simulink model "Simscape_Benchmark_Model"  (R2020b)
settings: Solver=ode45  StartTime=0.0  StopTime=10.0  RelTol=1e-8  AbsTol=1e-9
undefined symbols (not defined in the file): Bus, FSM, ISOL, Model, PMA, RWIsol, RWS, SA, SADM, slosh, X, Y, Z
libraries: sm_lib x159, nesl_utility x85, simulink x4
(part 5 of 6)

== system Simscape_Benchmark_Model/WEMS + Reaction wheels/RW saturation and friction model ==
  note: 1) Add Subsystem or Model blocks as valid variant choices.
      | 2) You cannot connect blocks at this level. At simulation, connectivity is automatically
      | determined, based on the active variant and port name matching.
  In1 : Inport
  No saturations - No friction model : Subsystem  VariantControl=Benchmark.config.status.RWS_Sat==0 && Benchmark.config.status.RWS_Fric==0 && Benchmark.config.status.RWS_Frict_spikes==0
  Saturations +  friction model : Subsystem  VariantControl=Benchmark.config.status.RWS_Sat==1 && Benchmark.config.status.RWS_Fric==1 && Benchmark.config.status.RWS_Frict_spikes==0
  Saturations + friction model + friction spikes : Subsystem  VariantControl=Benchmark.config.status.RWS_Sat==1 && Benchmark.config.status.RWS_Fric==1 && Benchmark.config.status.RWS_Frict_spikes==1
  Saturations - No friction model : Subsystem  VariantControl=Benchmark.config.status.RWS_Sat==1 && Benchmark.config.status.RWS_Fric==0 && Benchmark.config.status.RWS_Frict_spikes==0
  Out1 : Outport

== system Simscape_Benchmark_Model/WEMS + Reaction wheels/RWS ==
  note: 1) Add Subsystem or Model blocks as valid variant choices.
      | 2) You cannot connect blocks at this level. At simulation, connectivity is automatically
      | determined, based on the active variant and port name matching.
  Balanced RWS : Subsystem  VariantControl="Benchmark.config.status.RWS_Harmdist==   0"
  RWS with disturbance harmonics : Subsystem  VariantControl="Benchmark.config.status.RWS_Harmdist==   1"
  Connection Port : PMIOPort  Tag=PMCPort  Side=Left
  Connection Port1 : PMIOPort  Tag=PMCPort  Port=2  Side=Left
  Connection Port2 : PMIOPort  Tag=PMCPort  Port=3  Side=Left
  Connection Port3 : PMIOPort  Tag=PMCPort  Port=4  Side=Left

== system Simscape_Benchmark_Model/WEMS + Reaction wheels/RW saturation and friction model/No saturations - No friction model ==
  In1 : Inport
  Out1 : Outport
  wires:
  In1/1 -> Out1/1

== system Simscape_Benchmark_Model/WEMS + Reaction wheels/RW saturation and friction model/Saturations +  friction model ==
  In1 : Inport
  RW friction model : Subsystem
  Terminator2 : Terminator
  sat_max_torque : Saturate  UpperLimit=RWS.max_torque  LowerLimit=-RWS.max_torque
  Out1 : Outport
  wires:
  In1/1 -> sat_max_torque/1
  sat_max_torque/1 -> RW friction model/1(Trq_cmd_rw)
  RW friction model/1(Torque_RW) -> Out1/1
  RW friction model/2(RW_TRQfriction) -> Terminator2/1

== system Simscape_Benchmark_Model/WEMS + Reaction wheels/RW saturation and friction model/Saturations + friction model + friction spikes ==
  In1 : Inport
  Gain : Gain  Gain=-1
  Mux : Mux
  Product : Product
  RW friction model : Subsystem
  Rate Transition : RateTransition  OutPortSampleTime=Model.ACS_sampling.Ts
  Spike generation RW1 : Subsystem
  Spike generation RW2 : Subsystem
  Spike generation RW3 : Subsystem
  Spike generation RW4 : Subsystem
  Sum : Sum
  Terminator2 : Terminator
  sat_max_torque : Saturate  UpperLimit=RWS.max_torque  LowerLimit=-RWS.max_torque
  Out1 : Outport
  tag scope: RW_torque_spikes=global
  wires:
  In1/1 -> sat_max_torque/1
  Sum/1 -> Out1/1
  Mux/1 -> Rate Transition/1
  RW friction model/1(Torque_RW) -> Sum/1
  RW friction model/2(RW_TRQfriction) -> Terminator2/1
  sat_max_torque/1 -> RW friction model/1(Trq_cmd_rw)
  Spike generation RW1/1(Out1) -> Mux/1
  Spike generation RW3/1(Out1) -> Mux/3
  Spike generation RW2/1(Out1) -> Mux/2
  Spike generation RW4/1(Out1) -> Mux/4
  RW friction model/3(sign_omega) -> Product/1
  Rate Transition/1 -> Gain/1
  Product/1 -> [RW_torque_spikes], Sum/2
  Gain/1 -> Product/2

== system Simscape_Benchmark_Model/WEMS + Reaction wheels/RW saturation and friction model/Saturations - No friction model ==
  In1 : Inport
  sat_max_torque : Saturate  UpperLimit=RWS.max_torque  LowerLimit=-RWS.max_torque
  Out1 : Outport
  wires:
  In1/1 -> sat_max_torque/1
  sat_max_torque/1 -> Out1/1

== system Simscape_Benchmark_Model/WEMS + Reaction wheels/RWS/Balanced RWS ==
  Cylindrical Solid{,1..3} (4 alike) : sm_lib/Body Elements/Cylindrical Solid  GraphicAmbientColor=[0.15 0.15 0.15 1.0]  BasedOnType=Density  CenterOfMass=[0 0 0]  CenterOfMassUnits=m  GraphicDiffuseColor=[0.8 0.0 0.0]  CylinderLength=0.1  CylinderLengthUnits=m  CylinderRadius=0.15  CylinderRadiusUnits=m  Density=1000  DensityUnits=kg/m^3  DoExposeReferenceFrame=on  GraphicEmissiveColor=[0.0 0.0 0.0 1.0]  ExportEntireGeometry=off  SerializedFrames=<Frames/>  MarkerShape=Sphere  MarkerSize=10  GraphicType=FromGeometry  InertiaType=Custom  Mass=RWS.m  MassUnits=kg  MomentsOfInertia=[RWS.Ir RWS.Ir RWS.Iw]  MomentsOfInertiaUnits=kg*m^2  GraphicOpacity=0.8  ProductsOfInertia=[0 0 0]  ProductsOfInertiaUnits=kg*m^2  GraphicShininess=75  GraphicSpecularColor=[0.5 0.5 0.5 1.0]  GraphicVisPropType=SimpleVisualProperties
  Frame R_RW{1..4} (4 alike) : sm_lib/Body Elements/Graphic  GraphicType=Marker  MarkerShape=Frame  MarkerSize=35  GraphicVisPropType=SimpleVisualProperties  GraphicDiffuseColor=[0.2 1.0 1.0]  GraphicSpecularColor=[0.5 0.5 0.5 1.0]  GraphicAmbientColor=[0.15 0.15 0.15 1.0]  GraphicEmissiveColor=[0.0 0.0 0.0 1.0]  GraphicShininess=75  GraphicOpacity=0.5
  Connection Port : PMIOPort  Tag=PMCPort  Side=Left
  Connection Port1 : PMIOPort  Tag=PMCPort  Port=2  Side=Left
  Connection Port2 : PMIOPort  Tag=PMCPort  Port=3  Side=Left
  Connection Port3 : PMIOPort  Tag=PMCPort  Port=4  Side=Left
  connections:
  Frame R_RW1/RConn1 -- Connection Port/RConn1 -- Cylindrical Solid/RConn1
  Cylindrical Solid1/RConn1 -- Connection Port1/RConn1 -- Frame R_RW2/RConn1
  Cylindrical Solid2/RConn1 -- Connection Port2/RConn1 -- Frame R_RW3/RConn1
  Cylindrical Solid3/RConn1 -- Connection Port3/RConn1 -- Frame R_RW4/RConn1

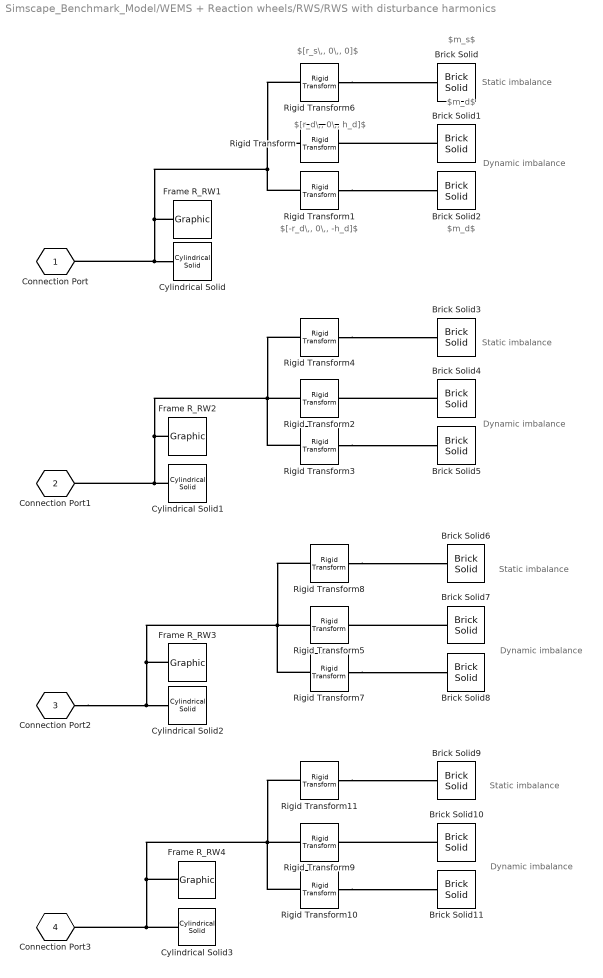
== system Simscape_Benchmark_Model/WEMS + Reaction wheels/RWS/RWS with disturbance harmonics ==
  note: Static imbalance
  note: Dynamic imbalance
  note: Static imbalance
  note: Dynamic imbalance
  note: Static imbalance
  note: Dynamic imbalance
  note: Static imbalance
  note: Dynamic imbalance
  note: $[r_s\,, 0\,, 0]$
  note: $m_s$
  note: $[r_d\,, 0\,, h_d]$
  note: $m_d$
  note: $[-r_d\,, 0\,, -h_d]$
  note: $m_d$
  Brick Solid{,3,6,9} (4 alike) : sm_lib/Body Elements/Brick Solid  GraphicAmbientColor=[0.15 0.15 0.15 1.0]  BasedOnType=Density  BrickDimensions=[0.01 0.01 0.01]  BrickDimensionUnits=m  CenterOfMass=[0 0 0]  CenterOfMassUnits=m  GraphicDiffuseColor=[0.5 0.5 0.5]  Density=1000  DensityUnits=kg/m^3  DoExposeReferenceFrame=on  GraphicEmissiveColor=[0.0 0.0 0.0 1.0]  ExportEntireGeometry=off  SerializedFrames=<Frames/>  MarkerShape=Sphere  MarkerSize=10  GraphicType=None  InertiaType=PointMass  Mass=RWS.m_s  MassUnits=kg  MomentsOfInertia=[1 1 1]  MomentsOfInertiaUnits=kg*m^2  GraphicOpacity=1.0  ProductsOfInertia=[0 0 0]  ProductsOfInertiaUnits=kg*m^2  GraphicShininess=75  GraphicSpecularColor=[0.5 0.5 0.5 1.0]  GraphicVisPropType=SimpleVisualProperties
  Brick Solid{1..2,4..5,7..8,10..11} (8 alike) : sm_lib/Body Elements/Brick Solid  GraphicAmbientColor=[0.15 0.15 0.15 1.0]  BasedOnType=Density  BrickDimensions=[0.01 0.01 0.01]  BrickDimensionUnits=m  CenterOfMass=[0 0 0]  CenterOfMassUnits=m  GraphicDiffuseColor=[0.5 0.5 0.5]  Density=1000  DensityUnits=kg/m^3  DoExposeReferenceFrame=on  GraphicEmissiveColor=[0.0 0.0 0.0 1.0]  ExportEntireGeometry=off  SerializedFrames=<Frames/>  MarkerShape=Sphere  MarkerSize=10  GraphicType=None  InertiaType=PointMass  Mass=RWS.m_d  MassUnits=kg  MomentsOfInertia=[1 1 1]  MomentsOfInertiaUnits=kg*m^2  GraphicOpacity=1.0  ProductsOfInertia=[0 0 0]  ProductsOfInertiaUnits=kg*m^2  GraphicShininess=75  GraphicSpecularColor=[0.5 0.5 0.5 1.0]  GraphicVisPropType=SimpleVisualProperties
  Cylindrical Solid{,1..3} (4 alike) : sm_lib/Body Elements/Cylindrical Solid  GraphicAmbientColor=[0.15 0.15 0.15 1.0]  BasedOnType=Density  CenterOfMass=[0 0 0]  CenterOfMassUnits=m  GraphicDiffuseColor=[0.5 0.5 0.5]  CylinderLength=0.1  CylinderLengthUnits=m  CylinderRadius=0.15  CylinderRadiusUnits=m  Density=1000  DensityUnits=kg/m^3  DoExposeReferenceFrame=on  GraphicEmissiveColor=[0.0 0.0 0.0 1.0]  ExportEntireGeometry=off  SerializedFrames=<Frames/>  MarkerShape=Sphere  MarkerSize=10  GraphicType=FromGeometry  InertiaType=Custom  Mass=RWS.m  MassUnits=kg  MomentsOfInertia=[RWS.Ir RWS.Ir RWS.Iw]  MomentsOfInertiaUnits=kg*m^2  GraphicOpacity=1.0  ProductsOfInertia=[0 0 0]  ProductsOfInertiaUnits=kg*m^2  GraphicShininess=75  GraphicSpecularColor=[0.5 0.5 0.5 1.0]  GraphicVisPropType=SimpleVisualProperties
  Frame R_RW1 : sm_lib/Body Elements/Graphic  GraphicType=Marker  MarkerShape=Frame  MarkerSize=45  GraphicVisPropType=SimpleVisualProperties  GraphicDiffuseColor=[0.2 1.0 1.0]  GraphicSpecularColor=[0.5 0.5 0.5 1.0]  GraphicAmbientColor=[0.15 0.15 0.15 1.0]  GraphicEmissiveColor=[0.0 0.0 0.0 1.0]  GraphicShininess=75  GraphicOpacity=1.0
  Frame R_RW2 : sm_lib/Body Elements/Graphic  GraphicType=Marker  MarkerShape=Frame  MarkerSize=25  GraphicVisPropType=SimpleVisualProperties  GraphicDiffuseColor=[0.2 1.0 1.0]  GraphicSpecularColor=[0.5 0.5 0.5 1.0]  GraphicAmbientColor=[0.15 0.15 0.15 1.0]  GraphicEmissiveColor=[0.0 0.0 0.0 1.0]  GraphicShininess=75  GraphicOpacity=1.0
  Frame R_RW3 : sm_lib/Body Elements/Graphic  GraphicType=Marker  MarkerShape=Frame  MarkerSize=50  GraphicVisPropType=SimpleVisualProperties  GraphicDiffuseColor=[0.2 1.0 1.0]  GraphicSpecularColor=[0.5 0.5 0.5 1.0]  GraphicAmbientColor=[0.15 0.15 0.15 1.0]  GraphicEmissiveColor=[0.0 0.0 0.0 1.0]  GraphicShininess=75  GraphicOpacity=1.0
  Frame R_RW4 : sm_lib/Body Elements/Graphic  GraphicType=Marker  MarkerShape=Frame  MarkerSize=25  GraphicVisPropType=SimpleVisualProperties  GraphicDiffuseColor=[0.2 1.0 1.0]  GraphicSpecularColor=[0.5 0.5 0.5 1.0]  GraphicAmbientColor=[0.15 0.15 0.15 1.0]  GraphicEmissiveColor=[0.0 0.0 0.0 1.0]  GraphicShininess=75  GraphicOpacity=1.0
  Rigid Transform{,2,5,9} (4 alike) : sm_lib/Frames and Transforms/Rigid Transform  TranslationMethod=Cartesian  TranslationStandardOffset=0  TranslationLengthUnit=m  TranslationStandardAxis=+Z  TranslationCartesianOffset=[RWS.r_d 0 RWS.h_d]  TranslationROffset=0  TranslationROffsetUnits=m  TranslationZOffset=0  TranslationZOffsetUnits=m  TranslationThetaOffset=0  TranslationThetaOffsetUnits=deg  RotationMethod=None  RotationAngleUnits=deg  RotationStandardAxis=+Z  RotationAngle=0.0  RotationArbitraryAxis=[0 0 1]  FollAlignAxisA=+X  BaseAlignAxisA=+Y  FollAlignAxisB=+Y  BaseAlignAxisB=+Z  RotationSequenceAxes=FollowerAxes  RotationSequence=XYX  RotationSequenceAngles=[0 0 0]  RotationSequenceAnglesUnits=deg  RotationMatrix=[1 0 0; 0 1 0; 0 0 1]
  Rigid Transform{1,3,7,10} (4 alike) : sm_lib/Frames and Transforms/Rigid Transform  TranslationMethod=Cartesian  TranslationStandardOffset=0  TranslationLengthUnit=m  TranslationStandardAxis=+Z  TranslationCartesianOffset=[-RWS.r_d 0 -RWS.h_d]  TranslationROffset=0  TranslationROffsetUnits=m  TranslationZOffset=0  TranslationZOffsetUnits=m  TranslationThetaOffset=0  TranslationThetaOffsetUnits=deg  RotationMethod=None  RotationAngleUnits=deg  RotationStandardAxis=+Z  RotationAngle=0.0  RotationArbitraryAxis=[0 0 1]  FollAlignAxisA=+X  BaseAlignAxisA=+Y  FollAlignAxisB=+Y  BaseAlignAxisB=+Z  RotationSequenceAxes=FollowerAxes  RotationSequence=XYX  RotationSequenceAngles=[0 0 0]  RotationSequenceAnglesUnits=deg  RotationMatrix=[1 0 0; 0 1 0; 0 0 1]
  Rigid Transform{4,6,8,11} (4 alike) : sm_lib/Frames and Transforms/Rigid Transform  TranslationMethod=Cartesian  TranslationStandardOffset=0  TranslationLengthUnit=m  TranslationStandardAxis=+Z  TranslationCartesianOffset=[RWS.r_s 0 0]  TranslationROffset=0  TranslationROffsetUnits=m  TranslationZOffset=0  TranslationZOffsetUnits=m  TranslationThetaOffset=0  TranslationThetaOffsetUnits=deg  RotationMethod=None  RotationAngleUnits=deg  RotationStandardAxis=+Z  RotationAngle=0.0  RotationArbitraryAxis=[0 0 1]  FollAlignAxisA=+X  BaseAlignAxisA=+Y  FollAlignAxisB=+Y  BaseAlignAxisB=+Z  RotationSequenceAxes=FollowerAxes  RotationSequence=XYX  RotationSequenceAngles=[0 0 0]  RotationSequenceAnglesUnits=deg  RotationMatrix=[1 0 0; 0 1 0; 0 0 1]
  Connection Port : PMIOPort  Tag=PMCPort  Side=Left
  Connection Port1 : PMIOPort  Tag=PMCPort  Port=2  Side=Left
  Connection Port2 : PMIOPort  Tag=PMCPort  Port=3  Side=Left
  Connection Port3 : PMIOPort  Tag=PMCPort  Port=4  Side=Left
  connections:
  Brick Solid1/RConn1 -- Rigid Transform/RConn1
  Rigid Transform1/RConn1 -- Brick Solid2/RConn1
  Rigid Transform6/RConn1 -- Brick Solid/RConn1
  Rigid Transform1/LConn1 -- Frame R_RW1/RConn1 -- Connection Port/RConn1 -- Cylindrical Solid/RConn1 -- Rigid Transform6/LConn1 -- Rigid Transform/LConn1
  Rigid Transform2/LConn1 -- Rigid Transform4/LConn1 -- Rigid Transform3/LConn1 -- Connection Port1/RConn1 -- Cylindrical Solid1/RConn1 -- Frame R_RW2/RConn1
  Rigid Transform5/LConn1 -- Rigid Transform8/LConn1 -- Rigid Transform7/LConn1 -- Connection Port2/RConn1 -- Cylindrical Solid2/RConn1 -- Frame R_RW3/RConn1
  Rigid Transform9/LConn1 -- Frame R_RW4/RConn1 -- Cylindrical Solid3/RConn1 -- Connection Port3/RConn1 -- Rigid Transform11/LConn1 -- Rigid Transform10/LConn1
  Rigid Transform3/RConn1 -- Brick Solid5/RConn1
  Brick Solid4/RConn1 -- Rigid Transform2/RConn1
  Rigid Transform4/RConn1 -- Brick Solid3/RConn1
  Rigid Transform8/RConn1 -- Brick Solid6/RConn1
  Rigid Transform7/RConn1 -- Brick Solid8/RConn1
  Brick Solid7/RConn1 -- Rigid Transform5/RConn1
  Rigid Transform10/RConn1 -- Brick Solid11/RConn1
  Brick Solid10/RConn1 -- Rigid Transform9/RConn1
  Rigid Transform11/RConn1 -- Brick Solid9/RConn1

== system Simscape_Benchmark_Model/WEMS + Reaction wheels/RW saturation and friction model/Saturations +  friction model/RW friction model ==
  Trq_cmd_rw : Inport
  Friction model (torque) : Subsystem
  Mux : Mux
  Rate Transition : RateTransition  OutPortSampleTime=Model.ACS_sampling.Ts
  Torque_RW : Outport
  RW_TRQfriction : Outport  Port=2  VectorParamsAs1DForOutWhenUnconnected=off
  tag scope: RW_Friction=global
  wires:
  [RW4_speed] -> Mux/4
  Mux/1 -> Rate Transition/1
  Trq_cmd_rw/1 -> Friction model (torque)/2(motor cmd trq (Nm))
  Friction model (torque)/2(Torque_friction) -> [RW_Friction], RW_TRQfriction/1  "rw_Trqfriction"
  [RW2_speed] -> Mux/2
  [RW3_speed] -> Mux/3
  [RW1_speed] -> Mux/1
  Rate Transition/1 -> Friction model (torque)/1(rw_speed (rad/s))
  Friction model (torque)/1(Torque_total) -> Torque_RW/1

== system Simscape_Benchmark_Model/WEMS + Reaction wheels/RW saturation and friction model/Saturations + friction model + friction spikes/RW friction model ==
  Trq_cmd_rw : Inport
  Friction model (torque)1 : Subsystem
  Mux : Mux
  Rate Transition : RateTransition  OutPortSampleTime=Model.ACS_sampling.Ts
  Torque_RW : Outport
  RW_TRQfriction : Outport  Port=2  VectorParamsAs1DForOutWhenUnconnected=off
  sign_omega : Outport  Port=3
  tag scope: RW_Friction=global
  wires:
  [RW4_speed] -> Mux/4
  Mux/1 -> Rate Transition/1
  Trq_cmd_rw/1 -> Friction model (torque)1/2(motor cmd trq (Nm))
  Friction model (torque)1/2(Torque_friction) -> [RW_Friction], RW_TRQfriction/1  "rw_Trqfriction"
  [RW2_speed] -> Mux/2
  Friction model (torque)1/1(Torque_total) -> Torque_RW/1
  [RW3_speed] -> Mux/3
  [RW1_speed] -> Mux/1
  Rate Transition/1 -> Friction model (torque)1/1(rw_speed (rad/s))
  Friction model (torque)1/3(sign_omega) -> sign_omega/1

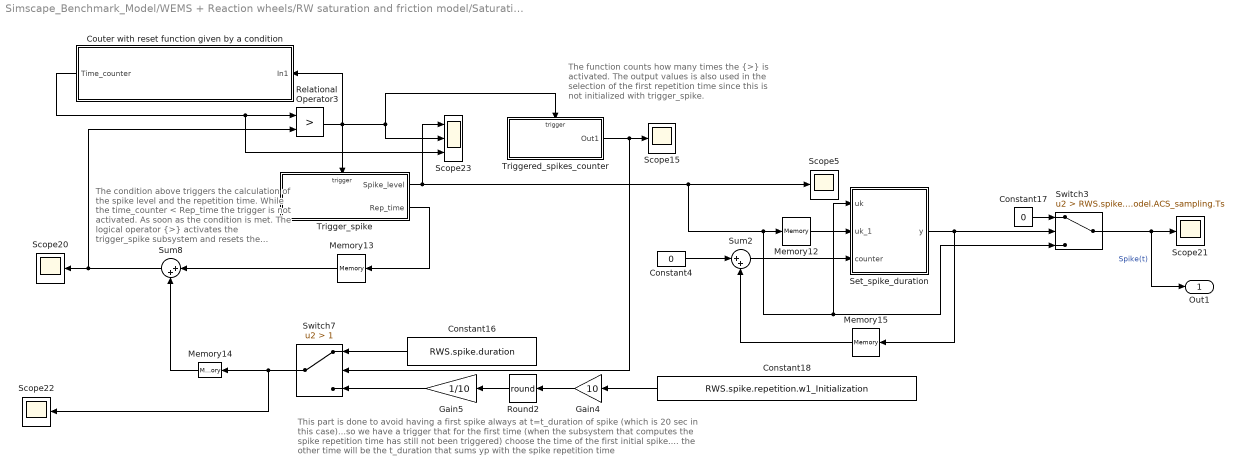
== system Simscape_Benchmark_Model/WEMS + Reaction wheels/RW saturation and friction model/Saturations + friction model + friction spikes/Spike generation RW1 ==
  note: The condition above triggers the calculation of the spike level and the repetition time.
      | While the time_counter < Rep_time the trigger is not activated. As soon as the condition is met. The logical operator {>} activates the trigger_spike subsystem and resets the counter.
  note: The function counts how many times the {>} is activated. The output values is also used in the selection of the first repetition time since this is not initialized with trigger_spike.
  note: This part is done to avoid having a first spike always at t=t_duration of spike (which is 20 sec in this case)...so we have a trigger that for the first time (when the subsystem that computes the spike repetition time has still not been triggered) choose the time of the first initial spike.... the other time will be the t_duration that sums yp with the spike repetition time
  Constant16 : Constant  Value=RWS.spike.duration
  Constant17 : Constant  Value=0  SampleTime=Inf
  Constant18 : Constant  Value=RWS.spike.repetition.w1_Initialization  SampleTime=Inf
  Constant4 : Constant  Value=0  SampleTime=Inf
  Couter with reset function given by a condition : Subsystem
  Gain4 : Gain  Gain=10
  Gain5 : Gain  Gain=1/10
  Memory12 : Memory  InheritSampleTime=on
  Memory13 : Memory  InheritSampleTime=on
  Memory14 : Memory
  Memory15 : Memory  InheritSampleTime=on
  Relational Operator3 : RelationalOperator  Operator=>  OutDataTypeStr=boolean  RndMeth=Simplest
  Round2 : Rounding  Operator=round
  Scope{5,15,20..22} (5 alike) : Scope
  Scope23 : Scope  NumInputPorts=3
  Set_spike_duration : MATLAB Function  TreatAsAtomicUnit=on
  Sum2 : Sum  Inputs=|++
  Sum8 : Sum  Inputs=|++
  Switch3 : Switch  Criteria=u2 > Threshold  Threshold=RWS.spike.duration/Model.ACS_sampling.Ts
  Switch7 : Switch  Criteria=u2 > Threshold  Threshold=1
  Trigger_spike : Subsystem  TreatAsAtomicUnit=on
  Triggered_spikes_counter : Subsystem  TreatAsAtomicUnit=on
  Out1 : Outport
  wires:
  Constant16/1 -> Switch7/1
  Sum8/1 -> Relational Operator3/2, Scope20/1
  Gain5/1 -> Switch7/3
  Set_spike_duration/1(y) -> Switch3/2, Memory15/1
  Relational Operator3/1 -> Scope23/2, Triggered_spikes_counter/Trigger, Couter with reset function given by a condition/1(In1), Trigger_spike/Trigger
  Constant18/1 -> Gain4/1
  Sum2/1 -> Set_spike_duration/3(counter)
  Constant4/1 -> Sum2/1
  Round2/1 -> Gain5/1
  Memory12/1 -> Set_spike_duration/2(uk_1)
  Memory13/1 -> Sum8/1
  Trigger_spike/1(Spike_level) -> Set_spike_duration/1(uk), Switch3/3, Memory12/1, Scope5/1, Scope23/1
  Memory14/1 -> Sum8/2
  Trigger_spike/2(Rep_time) -> Memory13/1
  Switch3/1 -> Out1/1, Scope21/1  "Spike(t)"
  Constant17/1 -> Switch3/1
  Memory15/1 -> Sum2/2
  Triggered_spikes_counter/1(Out1) -> Scope15/1, Switch7/2
  Gain4/1 -> Round2/1
  Couter with reset function given by a condition/1(Time_counter) -> Relational Operator3/1, Scope23/3
  Switch7/1 -> Scope22/1, Memory14/1

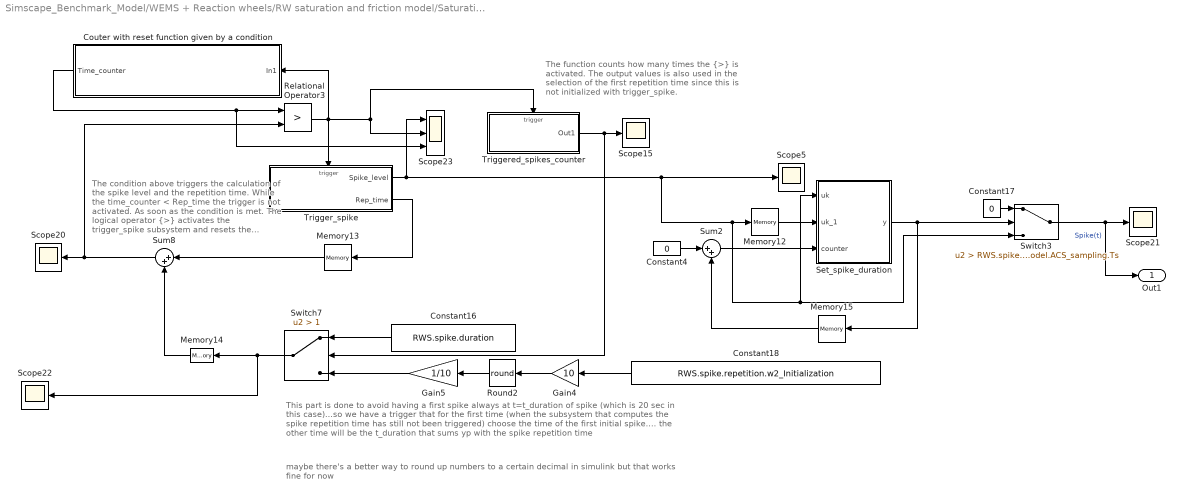
== system Simscape_Benchmark_Model/WEMS + Reaction wheels/RW saturation and friction model/Saturations + friction model + friction spikes/Spike generation RW2 ==
  note: The condition above triggers the calculation of the spike level and the repetition time.
      | While the time_counter < Rep_time the trigger is not activated. As soon as the condition is met. The logical operator {>} activates the trigger_spike subsystem and resets the counter.
  note: maybe there's a better way to round up numbers to a certain decimal in simulink but that works fine for now
  note: The function counts how many times the {>} is activated. The output values is also used in the selection of the first repetition time since this is not initialized with trigger_spike.
  note: This part is done to avoid having a first spike always at t=t_duration of spike (which is 20 sec in this case)...so we have a trigger that for the first time (when the subsystem that computes the spike repetition time has still not been triggered) choose the time of the first initial spike.... the other time will be the t_duration that sums yp with the spike repetition time
  Constant16 : Constant  Value=RWS.spike.duration
  Constant17 : Constant  Value=0  SampleTime=Model.ACS_sampling.Ts
  Constant18 : Constant  Value=RWS.spike.repetition.w2_Initialization  SampleTime=Inf
  Constant4 : Constant  Value=0  SampleTime=Model.ACS_sampling.Ts
  Couter with reset function given by a condition : Subsystem
  Gain4 : Gain  Gain=10
  Gain5 : Gain  Gain=1/10
  Memory{12..15} (4 alike) : Memory
  Relational Operator3 : RelationalOperator  Operator=>  OutDataTypeStr=boolean  RndMeth=Simplest
  Round2 : Rounding  Operator=round
  Scope{5,15,20..22} (5 alike) : Scope
  Scope23 : Scope  NumInputPorts=3
  Set_spike_duration : MATLAB Function  TreatAsAtomicUnit=on
  Sum2 : Sum  Inputs=|++
  Sum8 : Sum  Inputs=|++
  Switch3 : Switch  Criteria=u2 > Threshold  Threshold=RWS.spike.duration/Model.ACS_sampling.Ts
  Switch7 : Switch  Criteria=u2 > Threshold  Threshold=1
  Trigger_spike : Subsystem  TreatAsAtomicUnit=on
  Triggered_spikes_counter : Subsystem  TreatAsAtomicUnit=on
  Out1 : Outport
  wires:
  Constant16/1 -> Switch7/1
  Sum8/1 -> Relational Operator3/2, Scope20/1
  Gain5/1 -> Switch7/3
  Set_spike_duration/1(y) -> Switch3/2, Memory15/1
  Relational Operator3/1 -> Scope23/2, Triggered_spikes_counter/Trigger, Couter with reset function given by a condition/1(In1), Trigger_spike/Trigger
  Constant18/1 -> Gain4/1
  Sum2/1 -> Set_spike_duration/3(counter)
  Constant4/1 -> Sum2/1
  Round2/1 -> Gain5/1
  Memory12/1 -> Set_spike_duration/2(uk_1)
  Memory13/1 -> Sum8/1
  Trigger_spike/1(Spike_level) -> Set_spike_duration/1(uk), Switch3/3, Memory12/1, Scope5/1, Scope23/1
  Memory14/1 -> Sum8/2
  Trigger_spike/2(Rep_time) -> Memory13/1
  Switch3/1 -> Out1/1, Scope21/1  "Spike(t)"
  Constant17/1 -> Switch3/1
  Memory15/1 -> Sum2/2
  Triggered_spikes_counter/1(Out1) -> Scope15/1, Switch7/2
  Gain4/1 -> Round2/1
  Couter with reset function given by a condition/1(Time_counter) -> Relational Operator3/1, Scope23/3
  Switch7/1 -> Scope22/1, Memory14/1

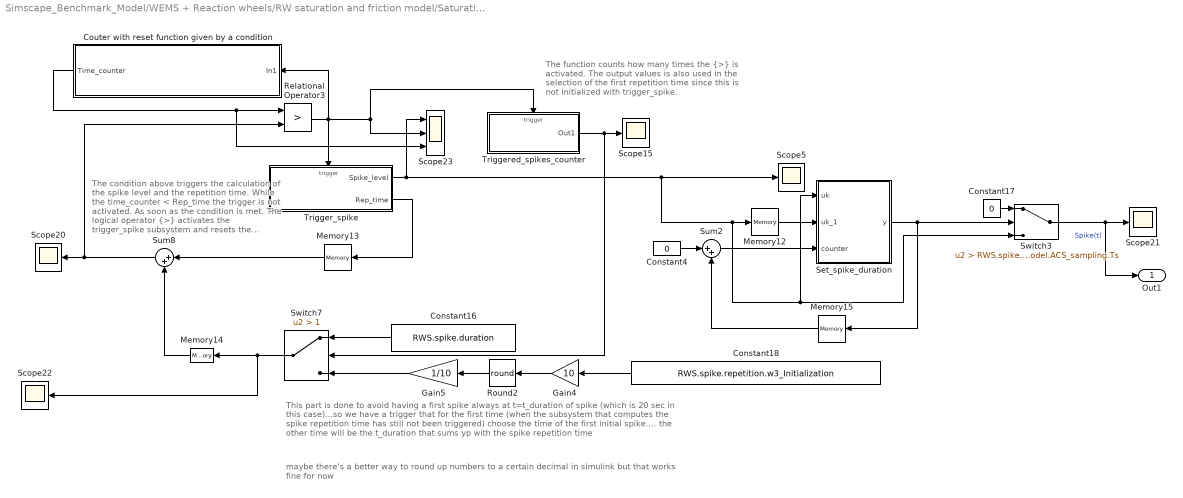
== system Simscape_Benchmark_Model/WEMS + Reaction wheels/RW saturation and friction model/Saturations + friction model + friction spikes/Spike generation RW3 ==
  note: The condition above triggers the calculation of the spike level and the repetition time.
      | While the time_counter < Rep_time the trigger is not activated. As soon as the condition is met. The logical operator {>} activates the trigger_spike subsystem and resets the counter.
  note: maybe there's a better way to round up numbers to a certain decimal in simulink but that works fine for now
  note: The function counts how many times the {>} is activated. The output values is also used in the selection of the first repetition time since this is not initialized with trigger_spike.
  note: This part is done to avoid having a first spike always at t=t_duration of spike (which is 20 sec in this case)...so we have a trigger that for the first time (when the subsystem that computes the spike repetition time has still not been triggered) choose the time of the first initial spike.... the other time will be the t_duration that sums yp with the spike repetition time
  Constant16 : Constant  Value=RWS.spike.duration
  Constant17 : Constant  Value=0  SampleTime=Model.ACS_sampling.Ts
  Constant18 : Constant  Value=RWS.spike.repetition.w3_Initialization  SampleTime=Inf
  Constant4 : Constant  Value=0  SampleTime=Model.ACS_sampling.Ts
  Couter with reset function given by a condition : Subsystem
  Gain4 : Gain  Gain=10
  Gain5 : Gain  Gain=1/10
  Memory{12..15} (4 alike) : Memory
  Relational Operator3 : RelationalOperator  Operator=>  OutDataTypeStr=boolean  RndMeth=Simplest
  Round2 : Rounding  Operator=round
  Scope{5,15,20..22} (5 alike) : Scope
  Scope23 : Scope  NumInputPorts=3
  Set_spike_duration : MATLAB Function  TreatAsAtomicUnit=on
  Sum2 : Sum  Inputs=|++
  Sum8 : Sum  Inputs=|++
  Switch3 : Switch  Criteria=u2 > Threshold  Threshold=RWS.spike.duration/Model.ACS_sampling.Ts
  Switch7 : Switch  Criteria=u2 > Threshold  Threshold=1
  Trigger_spike : Subsystem  TreatAsAtomicUnit=on
  Triggered_spikes_counter : Subsystem  TreatAsAtomicUnit=on
  Out1 : Outport
  wires:
  Constant16/1 -> Switch7/1
  Sum8/1 -> Relational Operator3/2, Scope20/1
  Gain5/1 -> Switch7/3
  Set_spike_duration/1(y) -> Switch3/2, Memory15/1
  Relational Operator3/1 -> Scope23/2, Triggered_spikes_counter/Trigger, Couter with reset function given by a condition/1(In1), Trigger_spike/Trigger
  Constant18/1 -> Gain4/1
  Sum2/1 -> Set_spike_duration/3(counter)
  Constant4/1 -> Sum2/1
  Round2/1 -> Gain5/1
  Memory12/1 -> Set_spike_duration/2(uk_1)
  Memory13/1 -> Sum8/1
  Trigger_spike/1(Spike_level) -> Set_spike_duration/1(uk), Switch3/3, Memory12/1, Scope5/1, Scope23/1
  Memory14/1 -> Sum8/2
  Trigger_spike/2(Rep_time) -> Memory13/1
  Switch3/1 -> Out1/1, Scope21/1  "Spike(t)"
  Constant17/1 -> Switch3/1
  Memory15/1 -> Sum2/2
  Triggered_spikes_counter/1(Out1) -> Scope15/1, Switch7/2
  Gain4/1 -> Round2/1
  Couter with reset function given by a condition/1(Time_counter) -> Relational Operator3/1, Scope23/3
  Switch7/1 -> Scope22/1, Memory14/1

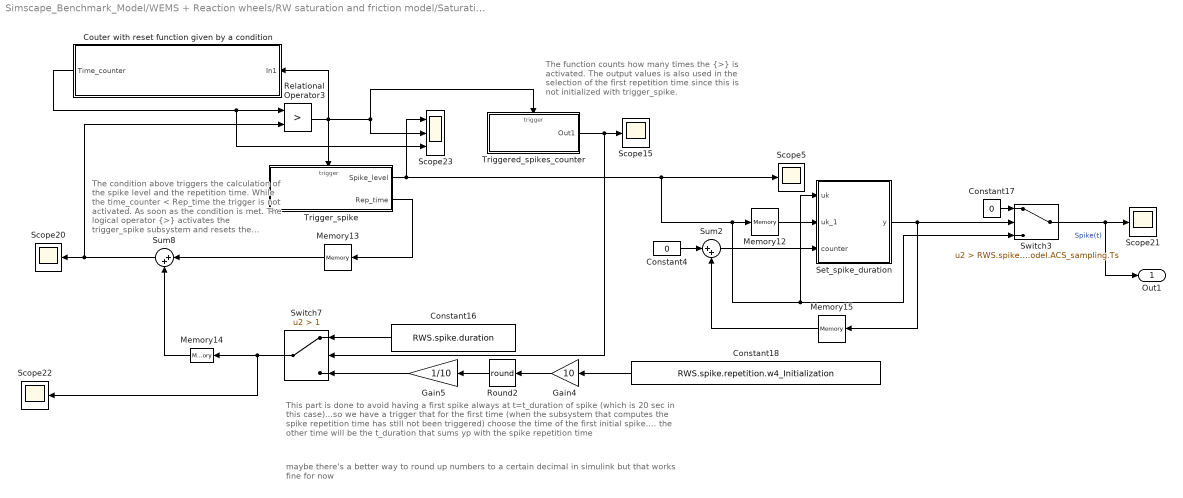
== system Simscape_Benchmark_Model/WEMS + Reaction wheels/RW saturation and friction model/Saturations + friction model + friction spikes/Spike generation RW4 ==
  note: The condition above triggers the calculation of the spike level and the repetition time.
      | While the time_counter < Rep_time the trigger is not activated. As soon as the condition is met. The logical operator {>} activates the trigger_spike subsystem and resets the counter.
  note: maybe there's a better way to round up numbers to a certain decimal in simulink but that works fine for now
  note: The function counts how many times the {>} is activated. The output values is also used in the selection of the first repetition time since this is not initialized with trigger_spike.
  note: This part is done to avoid having a first spike always at t=t_duration of spike (which is 20 sec in this case)...so we have a trigger that for the first time (when the subsystem that computes the spike repetition time has still not been triggered) choose the time of the first initial spike.... the other time will be the t_duration that sums yp with the spike repetition time
  Constant16 : Constant  Value=RWS.spike.duration
  Constant17 : Constant  Value=0  SampleTime=Model.ACS_sampling.Ts
  Constant18 : Constant  Value=RWS.spike.repetition.w4_Initialization  SampleTime=Inf
  Constant4 : Constant  Value=0  SampleTime=Model.ACS_sampling.Ts
  Couter with reset function given by a condition : Subsystem
  Gain4 : Gain  Gain=10
  Gain5 : Gain  Gain=1/10
  Memory{12..15} (4 alike) : Memory
  Relational Operator3 : RelationalOperator  Operator=>  OutDataTypeStr=boolean  RndMeth=Simplest
  Round2 : Rounding  Operator=round
  Scope{5,15,20..22} (5 alike) : Scope
  Scope23 : Scope  NumInputPorts=3
  Set_spike_duration : MATLAB Function  TreatAsAtomicUnit=on
  Sum2 : Sum  Inputs=|++
  Sum8 : Sum  Inputs=|++
  Switch3 : Switch  Criteria=u2 > Threshold  Threshold=RWS.spike.duration/Model.ACS_sampling.Ts
  Switch7 : Switch  Criteria=u2 > Threshold  Threshold=1
  Trigger_spike : Subsystem  TreatAsAtomicUnit=on
  Triggered_spikes_counter : Subsystem  TreatAsAtomicUnit=on
  Out1 : Outport
  wires:
  Constant16/1 -> Switch7/1
  Sum8/1 -> Relational Operator3/2, Scope20/1
  Gain5/1 -> Switch7/3
  Set_spike_duration/1(y) -> Switch3/2, Memory15/1
  Relational Operator3/1 -> Scope23/2, Triggered_spikes_counter/Trigger, Couter with reset function given by a condition/1(In1), Trigger_spike/Trigger
  Constant18/1 -> Gain4/1
  Sum2/1 -> Set_spike_duration/3(counter)
  Constant4/1 -> Sum2/1
  Round2/1 -> Gain5/1
  Memory12/1 -> Set_spike_duration/2(uk_1)
  Memory13/1 -> Sum8/1
  Trigger_spike/1(Spike_level) -> Set_spike_duration/1(uk), Switch3/3, Memory12/1, Scope5/1, Scope23/1
  Memory14/1 -> Sum8/2
  Trigger_spike/2(Rep_time) -> Memory13/1
  Switch3/1 -> Out1/1, Scope21/1  "Spike(t)"
  Constant17/1 -> Switch3/1
  Memory15/1 -> Sum2/2
  Triggered_spikes_counter/1(Out1) -> Scope15/1, Switch7/2
  Gain4/1 -> Round2/1
  Couter with reset function given by a condition/1(Time_counter) -> Relational Operator3/1, Scope23/3
  Switch7/1 -> Scope22/1, Memory14/1

== system Simscape_Benchmark_Model/WEMS + Reaction wheels/RW saturation and friction model/Saturations +  friction model/RW friction model/Friction model (torque) ==
  rw_speed (rad/s) : Inport
  motor cmd trq (Nm) : Inport  Port=2
  Computation of the sign of rw_speed : Subsystem
  Friction torque calculation : Subsystem
  Sum : Sum  Inputs=+++  SaturateOnIntegerOverflow=on
  Sum1 : Sum  SaturateOnIntegerOverflow=on
  Torque_total : Outport  VectorParamsAs1DForOutWhenUnconnected=off
  Torque_friction : Outport  Port=2  VectorParamsAs1DForOutWhenUnconnected=off
  wires:
  rw_speed (rad/s)/1 -> Computation of the sign of rw_speed/1(rw_speed), Friction torque calculation/1(rw_speed)
  Computation of the sign of rw_speed/1(sign_rw_speed) -> Friction torque calculation/2(sign_rw_speed)
  Friction torque calculation/2(Torque_stiction) -> Sum/2
  Friction torque calculation/1(Torque_Coulomb) -> Sum/1
  Sum1/1 -> Torque_total/1
  Friction torque calculation/3(Torque_viscous) -> Sum/3
  Sum/1 -> Torque_friction/1, Sum1/1
  motor cmd trq (Nm)/1 -> Computation of the sign of rw_speed/2(Torque_motor), Sum1/2

== system Simscape_Benchmark_Model/WEMS + Reaction wheels/RW saturation and friction model/Saturations + friction model + friction spikes/RW friction model/Friction model (torque)1 ==
  rw_speed (rad/s) : Inport
  motor cmd trq (Nm) : Inport  Port=2
  Computation of the sign of rw_speed : Subsystem
  Friction torque calculation : Subsystem
  Sum : Sum  Inputs=+++  SaturateOnIntegerOverflow=on
  Sum1 : Sum  SaturateOnIntegerOverflow=on
  Torque_total : Outport  VectorParamsAs1DForOutWhenUnconnected=off
  Torque_friction : Outport  Port=2  VectorParamsAs1DForOutWhenUnconnected=off
  sign_omega : Outport  Port=3
  wires:
  rw_speed (rad/s)/1 -> Computation of the sign of rw_speed/1(rw_speed), Friction torque calculation/1(rw_speed)
  Friction torque calculation/2(Torque_stiction) -> Sum/2
  Friction torque calculation/1(Torque_Coulomb) -> Sum/1
  Sum1/1 -> Torque_total/1
  Friction torque calculation/3(Torque_viscous) -> Sum/3
  Sum/1 -> Torque_friction/1, Sum1/1
  motor cmd trq (Nm)/1 -> Computation of the sign of rw_speed/2(Torque_motor), Sum1/2
  Computation of the sign of rw_speed/1(sign_rw_speed) -> sign_omega/1, Friction torque calculation/2(sign_rw_speed)

== system Simscape_Benchmark_Model/WEMS + Reaction wheels/RW saturation and friction model/Saturations + friction model + friction spikes/Spike generation RW1/Couter with reset function given by a condition ==
  note: When the IF condition of the switch is met the counter gets reset at zero
  In1 : Inport
  Constant10 : Constant  SampleTime=Model.ACS_sampling.Ts
  Constant12 : Constant  Value=0  SampleTime=Model.ACS_sampling.Ts
  Delay : Delay  DelayLength=1  SampleTime=Model.ACS_sampling.Ts
  Memory17 : Memory  InheritSampleTime=on
  Scope18 : Scope
  Sum7 : Sum  Inputs=|++
  Switch6 : Switch  Criteria=u2 > Threshold
  Ts : Gain  Gain=Model.ACS_sampling.Ts
  Time_counter : Outport
  wires:
  Sum7/1 -> Switch6/3
  Constant10/1 -> Ts/1
  Ts/1 -> Sum7/1
  Constant12/1 -> Switch6/1
  Switch6/1 -> Delay/1, Time_counter/1, Scope18/1
  In1/1 -> Memory17/1
  Memory17/1 -> Switch6/2
  Delay/1 -> Sum7/2

== system Simscape_Benchmark_Model/WEMS + Reaction wheels/RW saturation and friction model/Saturations + friction model + friction spikes/Spike generation RW1/Trigger_spike ==
  note: way to round up at first decimal term
  Trigger : TriggerPort  VariantControl=Variant
  Constant : Constant  Value=RWS.spike.level.bias
  Constant1 : Constant  Value=RWS.spike.repetition.bias
  Gain : Gain  Gain=10
  Gain1 : Gain  Gain=1/10
  Gain2 : Gain  Gain=RWS.spike.level.scaling
  Gain3 : Gain  Gain=1/RWS.spike.level.rate
  Gain4 : Gain  Gain=1/RWS.spike.repetition.rate
  Gain5 : Gain  Gain=RWS.spike.mN2N
  Log : Math  Operator=log  SaturateOnIntegerOverflow=on
  Log2 : Math  Operator=log  SaturateOnIntegerOverflow=on
  Product : Product
  Round : Rounding  Operator=round
  Scope : Scope
  Sum : Sum  Inputs=-+
  Sum1 : Sum  Inputs=-+
  Uniform Random Number : UniformRandomNumber  Minimum=0  Seed=RWS.spike.w1seed(1)
  Uniform Random Number1 : UniformRandomNumber  Minimum=0  Seed=RWS.spike.w1seed(2)
  Uniform Random Number2 : UniformRandomNumber  Minimum=0  Seed=RWS.spike.w1seed(3)
  Spike_level : Outport
  Rep_time : Outport  Port=2
  wires:
  Gain2/1 -> Spike_level/1
  Sum1/1 -> Gain/1
  Gain1/1 -> Rep_time/1
  Gain/1 -> Round/1
  Round/1 -> Gain1/1
  Uniform Random Number/1 -> Product/1
  Uniform Random Number1/1 -> Product/2
  Constant/1 -> Sum/2
  Gain5/1 -> Gain2/1
  Product/1 -> Log/1
  Log/1 -> Gain3/1
  Gain3/1 -> Scope/1, Sum/1
  Gain4/1 -> Sum1/1
  Uniform Random Number2/1 -> Log2/1
  Constant1/1 -> Sum1/2
  Log2/1 -> Gain4/1
  Sum/1 -> Gain5/1

== system Simscape_Benchmark_Model/WEMS + Reaction wheels/RW saturation and friction model/Saturations + friction model + friction spikes/Spike generation RW1/Triggered_spikes_counter ==
  Trigger : TriggerPort  VariantControl=Variant
  Constant12 : Constant  Value=0
  Increment Stored Integer2 : simulink/Additional Math & Discrete/Additional Math: Increment - Decrement/Increment Stored Integer
  Sum8 : Sum
  Unit Delay1 : UnitDelay  SampleTime=-1  HasFrameUpgradeWarning=on
  Out1 : Outport
  wires:
  Constant12/1 -> Sum8/2
  Sum8/1 -> Increment Stored Integer2/1
  Unit Delay1/1 -> Sum8/1
  Increment Stored Integer2/1 -> Unit Delay1/1, Out1/1

== system Simscape_Benchmark_Model/WEMS + Reaction wheels/RW saturation and friction model/Saturations + friction model + friction spikes/Spike generation RW2/Couter with reset function given by a condition ==
  note: When the IF condition of the switch is met the counter gets reset at zero
  In1 : Inport
  Constant10 : Constant  SampleTime=Model.ACS_sampling.Ts
  Constant12 : Constant  Value=0  SampleTime=Model.ACS_sampling.Ts
  Delay : Delay  DelayLength=1  SampleTime=Model.ACS_sampling.Ts
  Memory17 : Memory
  Scope18 : Scope
  Sum7 : Sum  Inputs=|++
  Switch6 : Switch  Criteria=u2 > Threshold
  Ts : Gain  Gain=Model.ACS_sampling.Ts
  Time_counter : Outport
  wires:
  Sum7/1 -> Switch6/3
  Constant10/1 -> Ts/1
  Ts/1 -> Sum7/1
  Constant12/1 -> Switch6/1
  Switch6/1 -> Delay/1, Time_counter/1, Scope18/1
  In1/1 -> Memory17/1
  Memory17/1 -> Switch6/2
  Delay/1 -> Sum7/2

== system Simscape_Benchmark_Model/WEMS + Reaction wheels/RW saturation and friction model/Saturations + friction model + friction spikes/Spike generation RW2/Trigger_spike ==
  note: way to round up at first decimal term
  Trigger : TriggerPort  VariantControl=Variant
  Constant : Constant  Value=RWS.spike.level.bias
  Constant1 : Constant  Value=RWS.spike.repetition.bias
  Gain : Gain  Gain=10
  Gain1 : Gain  Gain=1/10
  Gain2 : Gain  Gain=RWS.spike.level.scaling
  Gain3 : Gain  Gain=1/RWS.spike.level.rate
  Gain4 : Gain  Gain=1/RWS.spike.repetition.rate
  Gain5 : Gain  Gain=RWS.spike.mN2N
  Log : Math  Operator=log  SaturateOnIntegerOverflow=on
  Log2 : Math  Operator=log  SaturateOnIntegerOverflow=on
  Product : Product
  Round : Rounding  Operator=round
  Scope : Scope
  Sum : Sum  Inputs=-+
  Sum1 : Sum  Inputs=-+
  Uniform Random Number : UniformRandomNumber  Minimum=0  Seed=RWS.spike.w2seed(1)
  Uniform Random Number1 : UniformRandomNumber  Minimum=0  Seed=RWS.spike.w2seed(2)
  Uniform Random Number2 : UniformRandomNumber  Minimum=0  Seed=RWS.spike.w2seed(3)
  Spike_level : Outport
  Rep_time : Outport  Port=2
  wires:
  Gain2/1 -> Spike_level/1
  Sum1/1 -> Gain/1
  Gain1/1 -> Rep_time/1
  Gain/1 -> Round/1
  Round/1 -> Gain1/1
  Uniform Random Number/1 -> Product/1
  Uniform Random Number1/1 -> Product/2
  Constant/1 -> Sum/2
  Gain5/1 -> Gain2/1
  Product/1 -> Log/1
  Log/1 -> Gain3/1
  Gain3/1 -> Scope/1, Sum/1
  Gain4/1 -> Sum1/1
  Uniform Random Number2/1 -> Log2/1
  Constant1/1 -> Sum1/2
  Log2/1 -> Gain4/1
  Sum/1 -> Gain5/1

== system Simscape_Benchmark_Model/WEMS + Reaction wheels/RW saturation and friction model/Saturations + friction model + friction spikes/Spike generation RW2/Triggered_spikes_counter ==
  Trigger : TriggerPort  VariantControl=Variant
  Constant12 : Constant  Value=0
  Increment Stored Integer2 : simulink/Additional Math & Discrete/Additional Math: Increment - Decrement/Increment Stored Integer
  Sum8 : Sum
  Unit Delay1 : UnitDelay  SampleTime=-1  HasFrameUpgradeWarning=on
  Out1 : Outport
  wires:
  Constant12/1 -> Sum8/2
  Sum8/1 -> Increment Stored Integer2/1
  Unit Delay1/1 -> Sum8/1
  Increment Stored Integer2/1 -> Unit Delay1/1, Out1/1

== system Simscape_Benchmark_Model/WEMS + Reaction wheels/RW saturation and friction model/Saturations + friction model + friction spikes/Spike generation RW3/Couter with reset function given by a condition ==
  note: When the IF condition of the switch is met the counter gets reset at zero
  In1 : Inport
  Constant10 : Constant  SampleTime=Model.ACS_sampling.Ts
  Constant12 : Constant  Value=0  SampleTime=Model.ACS_sampling.Ts
  Delay : Delay  DelayLength=1  SampleTime=Model.ACS_sampling.Ts
  Memory17 : Memory
  Scope18 : Scope
  Sum7 : Sum  Inputs=|++
  Switch6 : Switch  Criteria=u2 > Threshold
  Ts : Gain  Gain=Model.ACS_sampling.Ts
  Time_counter : Outport
  wires:
  Sum7/1 -> Switch6/3
  Constant10/1 -> Ts/1
  Ts/1 -> Sum7/1
  Constant12/1 -> Switch6/1
  Switch6/1 -> Delay/1, Time_counter/1, Scope18/1
  In1/1 -> Memory17/1
  Memory17/1 -> Switch6/2
  Delay/1 -> Sum7/2

== system Simscape_Benchmark_Model/WEMS + Reaction wheels/RW saturation and friction model/Saturations + friction model + friction spikes/Spike generation RW3/Trigger_spike ==
  note: way to round up at first decimal term
  Trigger : TriggerPort  VariantControl=Variant
  Constant : Constant  Value=RWS.spike.level.bias
  Constant1 : Constant  Value=RWS.spike.repetition.bias
  Gain : Gain  Gain=10
  Gain1 : Gain  Gain=1/10
  Gain2 : Gain  Gain=RWS.spike.level.scaling
  Gain3 : Gain  Gain=1/RWS.spike.level.rate
  Gain4 : Gain  Gain=1/RWS.spike.repetition.rate
  Gain5 : Gain  Gain=RWS.spike.mN2N
  Log : Math  Operator=log  SaturateOnIntegerOverflow=on
  Log2 : Math  Operator=log  SaturateOnIntegerOverflow=on
  Product : Product
  Round : Rounding  Operator=round
  Scope : Scope
  Sum : Sum  Inputs=-+
  Sum1 : Sum  Inputs=-+
  Uniform Random Number : UniformRandomNumber  Minimum=0  Seed=RWS.spike.w3seed(1)
  Uniform Random Number1 : UniformRandomNumber  Minimum=0  Seed=RWS.spike.w3seed(2)
  Uniform Random Number2 : UniformRandomNumber  Minimum=0  Seed=RWS.spike.w3seed(3)
  Spike_level : Outport
  Rep_time : Outport  Port=2
  wires:
  Gain2/1 -> Spike_level/1
  Sum1/1 -> Gain/1
  Gain1/1 -> Rep_time/1
  Gain/1 -> Round/1
  Round/1 -> Gain1/1
  Uniform Random Number/1 -> Product/1
  Uniform Random Number1/1 -> Product/2
  Constant/1 -> Sum/2
  Gain5/1 -> Gain2/1
  Product/1 -> Log/1
  Log/1 -> Gain3/1
  Gain3/1 -> Scope/1, Sum/1
  Gain4/1 -> Sum1/1
  Uniform Random Number2/1 -> Log2/1
  Constant1/1 -> Sum1/2
  Log2/1 -> Gain4/1
  Sum/1 -> Gain5/1

== system Simscape_Benchmark_Model/WEMS + Reaction wheels/RW saturation and friction model/Saturations + friction model + friction spikes/Spike generation RW3/Triggered_spikes_counter ==
  Trigger : TriggerPort  VariantControl=Variant
  Constant12 : Constant  Value=0
  Increment Stored Integer2 : simulink/Additional Math & Discrete/Additional Math: Increment - Decrement/Increment Stored Integer
  Sum8 : Sum
  Unit Delay1 : UnitDelay  SampleTime=-1  HasFrameUpgradeWarning=on
  Out1 : Outport
  wires:
  Constant12/1 -> Sum8/2
  Sum8/1 -> Increment Stored Integer2/1
  Unit Delay1/1 -> Sum8/1
  Increment Stored Integer2/1 -> Unit Delay1/1, Out1/1

== system Simscape_Benchmark_Model/WEMS + Reaction wheels/RW saturation and friction model/Saturations + friction model + friction spikes/Spike generation RW4/Couter with reset function given by a condition ==
  note: When the IF condition of the switch is met the counter gets reset at zero
  In1 : Inport
  Constant10 : Constant  SampleTime=Model.ACS_sampling.Ts
  Constant12 : Constant  Value=0  SampleTime=Model.ACS_sampling.Ts
  Delay : Delay  DelayLength=1  SampleTime=Model.ACS_sampling.Ts
  Memory17 : Memory
  Scope18 : Scope
  Sum7 : Sum  Inputs=|++
  Switch6 : Switch  Criteria=u2 > Threshold
  Ts : Gain  Gain=Model.ACS_sampling.Ts
  Time_counter : Outport
  wires:
  Sum7/1 -> Switch6/3
  Constant10/1 -> Ts/1
  Ts/1 -> Sum7/1
  Constant12/1 -> Switch6/1
  Switch6/1 -> Delay/1, Time_counter/1, Scope18/1
  In1/1 -> Memory17/1
  Memory17/1 -> Switch6/2
  Delay/1 -> Sum7/2

== system Simscape_Benchmark_Model/WEMS + Reaction wheels/RW saturation and friction model/Saturations + friction model + friction spikes/Spike generation RW4/Trigger_spike ==
  note: way to round up at first decimal term
  Trigger : TriggerPort  VariantControl=Variant
  Constant : Constant  Value=RWS.spike.level.bias
  Constant1 : Constant  Value=RWS.spike.repetition.bias
  Gain : Gain  Gain=10
  Gain1 : Gain  Gain=1/10
  Gain2 : Gain  Gain=RWS.spike.level.scaling
  Gain3 : Gain  Gain=1/RWS.spike.level.rate
  Gain4 : Gain  Gain=1/RWS.spike.repetition.rate
  Gain5 : Gain  Gain=RWS.spike.mN2N
  Log : Math  Operator=log  SaturateOnIntegerOverflow=on
  Log2 : Math  Operator=log  SaturateOnIntegerOverflow=on
  Product : Product
  Round : Rounding  Operator=round
  Scope : Scope
  Sum : Sum  Inputs=-+
  Sum1 : Sum  Inputs=-+
  Uniform Random Number : UniformRandomNumber  Minimum=0  Seed=RWS.spike.w4seed(1)
  Uniform Random Number1 : UniformRandomNumber  Minimum=0  Seed=RWS.spike.w4seed(2)
  Uniform Random Number2 : UniformRandomNumber  Minimum=0  Seed=RWS.spike.w4seed(3)
  Spike_level : Outport
  Rep_time : Outport  Port=2
  wires:
  Gain2/1 -> Spike_level/1
  Sum1/1 -> Gain/1
  Gain1/1 -> Rep_time/1
  Gain/1 -> Round/1
  Round/1 -> Gain1/1
  Uniform Random Number/1 -> Product/1
  Uniform Random Number1/1 -> Product/2
  Constant/1 -> Sum/2
  Gain5/1 -> Gain2/1
  Product/1 -> Log/1
  Log/1 -> Gain3/1
  Gain3/1 -> Scope/1, Sum/1
  Gain4/1 -> Sum1/1
  Uniform Random Number2/1 -> Log2/1
  Constant1/1 -> Sum1/2
  Log2/1 -> Gain4/1
  Sum/1 -> Gain5/1

== system Simscape_Benchmark_Model/WEMS + Reaction wheels/RW saturation and friction model/Saturations + friction model + friction spikes/Spike generation RW4/Triggered_spikes_counter ==
  Trigger : TriggerPort  VariantControl=Variant
  Constant12 : Constant  Value=0
  Increment Stored Integer2 : simulink/Additional Math & Discrete/Additional Math: Increment - Decrement/Increment Stored Integer
  Sum8 : Sum
  Unit Delay1 : UnitDelay  SampleTime=-1  HasFrameUpgradeWarning=on
  Out1 : Outport
  wires:
  Constant12/1 -> Sum8/2
  Sum8/1 -> Increment Stored Integer2/1
  Unit Delay1/1 -> Sum8/1
  Increment Stored Integer2/1 -> Unit Delay1/1, Out1/1

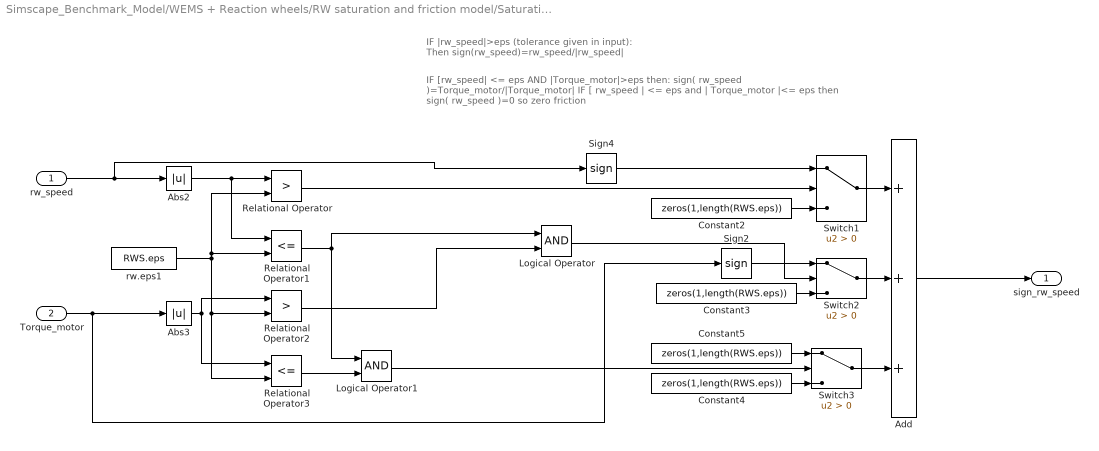
== system Simscape_Benchmark_Model/WEMS + Reaction wheels/RW saturation and friction model/Saturations +  friction model/RW friction model/Friction model (torque)/Computation of the sign of rw_speed ==
  note: IF [rw_speed| <= eps AND |Torque_motor|>eps then:
      | sign( rw_speed )=Torque_motor/|Torque_motor|
      |
      | IF [ rw_speed | <= eps and | Torque_motor |<= eps then sign( rw_speed )=0 so zero friction
  note: IF |rw_speed|>eps (tolerance given in input):
      | Then sign(rw_speed)=rw_speed/|rw_speed|
  rw_speed : Inport
  Torque_motor : Inport  Port=2
  Abs2 : Abs  SaturateOnIntegerOverflow=on
  Abs3 : Abs  SaturateOnIntegerOverflow=on
  Add : Sum  Inputs=+++
  Constant{2..5} (4 alike) : Constant  Value=zeros(1,length(RWS.eps))
  Logical Operator : Logic  AllPortsSameDT=off  OutDataTypeStr=boolean
  Logical Operator1 : Logic  AllPortsSameDT=off  OutDataTypeStr=boolean
  Relational Operator : RelationalOperator  Operator=>  OutDataTypeStr=boolean  ZeroCross=off  RndMeth=Nearest
  Relational Operator1 : RelationalOperator  Operator=<=  OutDataTypeStr=boolean  RndMeth=Nearest
  Relational Operator2 : RelationalOperator  Operator=>  OutDataTypeStr=boolean  ZeroCross=off  RndMeth=Nearest
  Relational Operator3 : RelationalOperator  Operator=<=  OutDataTypeStr=boolean  ZeroCross=off  RndMeth=Nearest
  Sign2 : Signum  ZeroCross=off
  Sign4 : Signum
  Switch1 : Switch  Criteria=u2 > Threshold  ZeroCross=off
  Switch2 : Switch  Criteria=u2 > Threshold  ZeroCross=off
  Switch3 : Switch  Criteria=u2 > Threshold  ZeroCross=off
  rw.eps1 : Constant  Value=RWS.eps
  sign_rw_speed : Outport  VectorParamsAs1DForOutWhenUnconnected=off
  wires:
  Logical Operator1/1 -> Switch3/2
  Logical Operator/1 -> Switch2/2
  Relational Operator3/1 -> Logical Operator1/2
  Relational Operator2/1 -> Logical Operator/2
  Abs3/1 -> Relational Operator3/1, Relational Operator2/1
  Relational Operator1/1 -> Logical Operator1/1, Logical Operator/1
  rw.eps1/1 -> Relational Operator/2, Relational Operator1/2, Relational Operator3/2, Relational Operator2/2
  Abs2/1 -> Relational Operator1/1, Relational Operator/1
  rw_speed/1 -> Sign4/1, Abs2/1
  Switch2/1 -> Add/2
  Constant5/1 -> Switch3/1
  Constant3/1 -> Switch2/3
  Sign4/1 -> Switch1/1
  Relational Operator/1 -> Switch1/2
  Switch1/1 -> Add/1
  Constant4/1 -> Switch3/3
  Constant2/1 -> Switch1/3
  Switch3/1 -> Add/3
  Sign2/1 -> Switch2/1
  Add/1 -> sign_rw_speed/1
  Torque_motor/1 -> Sign2/1, Abs3/1

== system Simscape_Benchmark_Model/WEMS + Reaction wheels/RW saturation and friction model/Saturations +  friction model/RW friction model/Friction model (torque)/Friction torque calculation ==
  note: IF |rw_speed|<=RWS.w_threshold then:
      |
      | Torque_stiction=-k_stiction*sign(rw_speed)
      |
      | otherwise Torque_stiction=0
  note: IF |rw_speed|>RWS.w_threshold then:
      |
      | Torque_Coulomb=-k_Coulomb*sign(rw_speed)
      |
      | otherwise Torque_Coulomb=0
  note: Torque_viscous=-k_viscous* rw_speed
  rw_speed : Inport
  sign_rw_speed : Inport  Port=2
  Abs : Abs  SaturateOnIntegerOverflow=on
  Gain : Gain  Gain=-1  SaturateOnIntegerOverflow=on  OutDataTypeStr=Inherit: Same as input  ParamDataTypeStr=Inherit: Same as input
  Gain1 : Gain  Gain=-1  SaturateOnIntegerOverflow=on  OutDataTypeStr=Inherit: Same as input  ParamDataTypeStr=Inherit: Same as input
  Gain2 : Gain  Gain=-1  SaturateOnIntegerOverflow=on  OutDataTypeStr=Inherit: Same as input  ParamDataTypeStr=Inherit: Same as input
  Switch : Switch  Threshold=RWS.w_threshold  ZeroCross=off  SaturateOnIntegerOverflow=on
  Switch2 : Switch  Threshold=RWS.w_threshold  ZeroCross=off  SaturateOnIntegerOverflow=on
  Torque_Coulomb=0 : Constant  Value=0
  Torque_stiction=0 : Constant  Value=0
  k_Coulomb : Gain  Gain=RWS.k_coulomb  SaturateOnIntegerOverflow=on  OutDataTypeStr=Inherit: Same as input  ParamDataTypeStr=Inherit: Same as input
  k_stiction : Gain  Gain=RWS.k_stiction  SaturateOnIntegerOverflow=on  OutDataTypeStr=Inherit: Same as input  ParamDataTypeStr=Inherit: Same as input
  k_viscous : Gain  Gain=RWS.k_viscous  SaturateOnIntegerOverflow=on  OutDataTypeStr=Inherit: Same as input  ParamDataTypeStr=Inherit: Same as input
  Torque_Coulomb : Outport  VectorParamsAs1DForOutWhenUnconnected=off
  Torque_stiction : Outport  Port=2  VectorParamsAs1DForOutWhenUnconnected=off
  Torque_viscous : Outport  Port=3  VectorParamsAs1DForOutWhenUnconnected=off
  wires:
  k_viscous/1 -> Torque_viscous/1
  Gain2/1 -> k_viscous/1
  Torque_stiction=0/1 -> Switch2/1
  k_stiction/1 -> Switch2/3
  Torque_Coulomb=0/1 -> Switch/3
  k_Coulomb/1 -> Switch/1
  Gain1/1 -> k_stiction/1
  Gain/1 -> k_Coulomb/1
  rw_speed/1 -> Gain2/1, Abs/1
  Abs/1 -> Switch2/2, Switch/2
  sign_rw_speed/1 -> Gain1/1, Gain/1
  Switch/1 -> Torque_Coulomb/1
  Switch2/1 -> Torque_stiction/1
